simulink model "vanderpol"  (R2025b)
settings: Solver=VariableStepAuto  StartTime=0.0  StopTime=50  RelTol=1e-3
settings Model: Creator=PC  LastModifiedBy=arabe
settings ModelReferenceCC: EnableRefExpFcnMdlSchedulingChecks=on
settings RTWCC: GPUComputeCapability=3.5

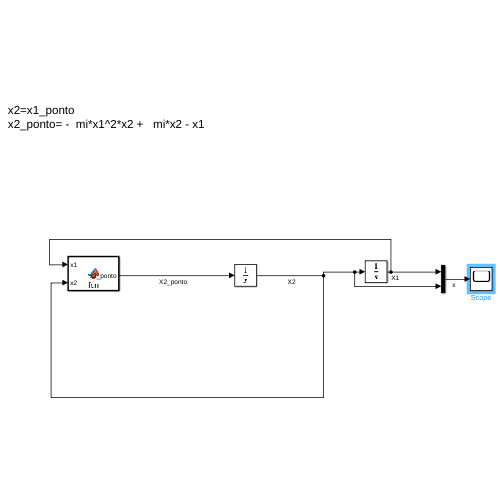
[thumbnail: Simulink's stored preview of the top-level diagram]
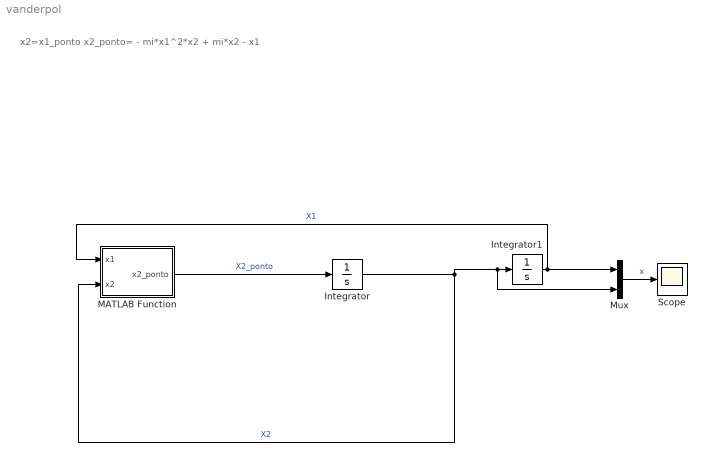
== system vanderpol ==
  note: x2=x1_ponto
      | x2_ponto= - mi*x1^2*x2 + mi*x2 - x1
  Integrator : Integrator
  Integrator1 : Integrator  InitialCondition=pi/2
  MATLAB Function : MATLAB Function  TreatAsAtomicUnit=on
  Mux : Mux  Inputs=2
  Scope : Scope
      settings: ActiveDisplayYMinimum=-3.34182  ActiveDisplayYMaximum=3.32477  DataLoggingSaveFormat=Array
  wires:
  Integrator1/1 -> MATLAB Function/1(x1), Mux/1  "X1"
  Mux/1 -> Scope/1  "x"
  Integrator/1 -> Mux/2, Integrator1/1, MATLAB Function/2(x2)  "X2"
  MATLAB Function/1(x2_ponto) -> Integrator/1  "X2_ponto"

== matlab function vanderpol/MATLAB Function ==
  data: x1 input; x2_ponto output; x2 input
function x2_ponto = fcn(x1,x2)

mi=1;
x2_ponto= -  mi*x1^2*x2 +   mi*x2 - x1;
